simulink model "inga_sima"  (Simulink 7.8)
settings: Solver=ode45  StartTime=0.0  StopTime=inf  RelTol=1e-3
values from neighbouring files (symbols this model uses):
  x1 = -pi:0.3:3*pi    [inga.m]
  x2 = -2:0.3:2    [inga.m]
libraries: vrlib x2
settings Model: Creator=valaki  LastModifiedBy=valaki

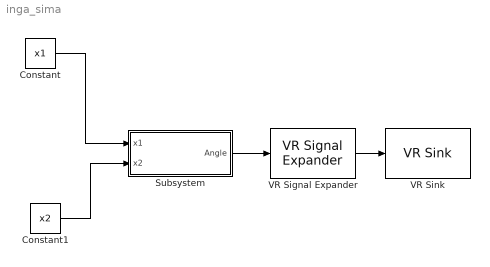
== system inga_sima ==
  Constant : Constant  Value=x1
  Constant1 : Constant  Value=x2
  Subsystem : Subsystem
  VR Signal Expander : vrlib/VR Signal Expander  outwidth=4  outidx=[4]
  VR Sink : vrlib/VR Sink  SampleTime=0.1  ViewEnable=on  RemoteChange=off  RemoteView=off  FieldsWritten=Ball.rotation.4.1.1.double  WorldFileName=C:\Users\valaki\Desktop\Pendulum_3D.wrl  WorldDescription=Forced Damped Pendulum  AutoView=off  VideoDimensions=[]  AllowVariableSize=off  FigureProperties="{'Position', 'Name', 'Viewpoint', 'CameraBound', 'CameraDirection', 'CameraPosition', 'CameraUpVector', 'ZoomFactor', 'Antialiasing', 'Headlight', 'Lighting', 'NavPanel', 'StatusBar', 'ToolBar', 'Textures', 'Transparency', 'Triad', 'Wireframe', 'NavZones', 'NavMode', 'NavSpeed', 'CaptureFileFormat', 'CaptureFileName', 'Record2DCompressMethod', 'Record2DCompressQuality', 'Record2D', 'Record2DFileName', 'Record2DFPS'; [2.1000000000000000e+001  1.2700000000000000e+002  5.7600000000000000e+002  3.8000000000000000e+002], 'Forced Damped Pendulum', 'Ball', 'on', [0.0000000000000000e+000  0.0000000000000000e+000 -1.0000000000000000e+000], [0.0000000000000000e+000  0.0000000000000000e+000  0.0000000000000000e+000], [0.0000000000000000e+000  1.0000000000000000e+000  0.0000000000000000e+000], [1.0000000000000000e+000], 'on', 'on', 'on', 'halfbar', 'on', 'on', 'on', 'on', 'none', 'off', 'off', 'walk', 'normal', 'tif', '%f_anim_%n.tif', 'auto', [7.5000000000000000e+001], 'off', '%f_anim_%n.avi', [1.5000000000000000e+001]}"
  wires:
  Constant/1 -> Subsystem/1(x1)
  Constant1/1 -> Subsystem/2(x2)
  Subsystem/1(Angle) -> VR Signal Expander/1
  VR Signal Expander/1 -> VR Sink/1

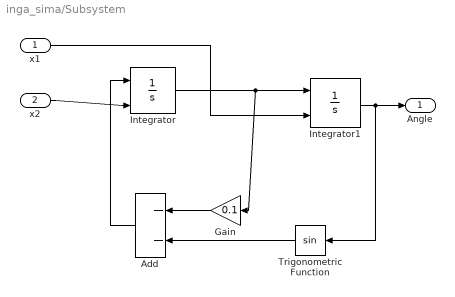
== system inga_sima/Subsystem ==
  x1 : Inport
  x2 : Inport  Port=2
  Add : Sum  Inputs=--
  Gain : Gain  Gain=0.1
  Integrator : Integrator  InitialConditionSource=external
  Integrator1 : Integrator  InitialConditionSource=external
  Trigonometric Function : Trigonometry
  Angle : Outport
  wires:
  x2/1 -> Integrator/2
  Integrator/1 -> Integrator1/1, Gain/1
  x1/1 -> Integrator1/2
  Integrator1/1 -> Angle/1, Trigonometric Function/1
  Add/1 -> Integrator/1
  Gain/1 -> Add/1
  Trigonometric Function/1 -> Add/2
